simulink model "UltrasonicDistanceSensor_7"  (R2023a)
settings: Solver=ode1  StartTime=0.0  StopTime=10.0  FixedStep=0.01  RelTol=1e-3
settings Model: Creator=MagneSirnes  LastModifiedBy=HalvorPlatou
settings DebuggingCC: UnconnectedInputMsg=warning  UnconnectedOutputMsg=warning  UnconnectedLineMsg=warning
settings ModelReferenceCC: EnableRefExpFcnMdlSchedulingChecks=on
settings RTWCC: DLArmComputeVersion=19.05

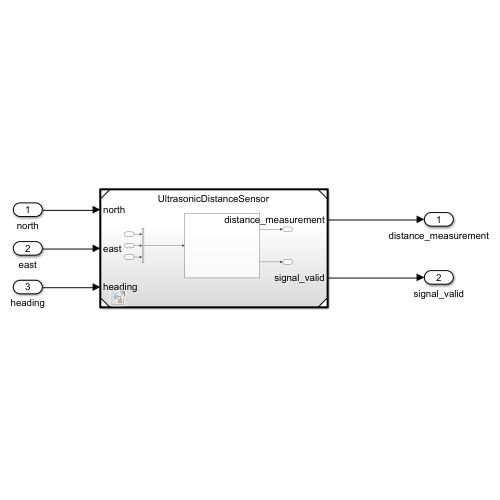
[thumbnail: Simulink's stored preview of the top-level diagram]
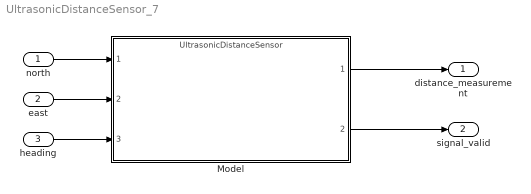
== system UltrasonicDistanceSensor_7 ==
  north : Inport  OutDataTypeStr=double
  east : Inport  Port=2  OutDataTypeStr=double
  heading : Inport  Port=3  OutDataTypeStr=double
  Model : ModelReference  ModelNameDialog=UltrasonicDistanceSensor.slx  SimulationMode=Normal  ModelReferenceVersion=2.1
  distance_measurement : Outport  OutDataTypeStr=double  PortDimensions=1
  signal_valid : Outport  Port=2  OutDataTypeStr=boolean  PortDimensions=1
  wires:
  north/1 -> Model/1
  east/1 -> Model/2
  heading/1 -> Model/3
  Model/2 -> signal_valid/1
  Model/1 -> distance_measurement/1
